simulink model "solverDiscStatesMultirate"  (R2022b)
settings: Solver=VariableStepDiscrete  StartTime=0.0  StopTime=20  RelTol=1e-3
settings Model: Creator=jrivitus  LastModifiedBy=bensweet
settings SolverCC: AlgebraicLoopSolver=TrustRegion
settings DataIOCC: LimitDataPoints=on  SaveFormat=Array  ReturnWorkspaceOutputs=off
settings OptimizationCC: ExpressionDepthLimit=2147483647  InitFltsAndDblsToZero=on  LifeSpan=inf
settings DebuggingCC: UnconnectedInputMsg=warning  UnconnectedOutputMsg=warning  UnconnectedLineMsg=warning  PregeneratedLibrarySubsystemCodeDiagnostic=none  SFMachineParentedDataDiag=warning
settings HardwareCC: ProdBitPerPointer=32  ProdBitPerSizeT=32  ProdBitPerPtrDiffT=32  ProdLargestAtomicFloat=None  ProdIntDivRoundTo=Undefined  ProdEndianess=Unspecified  ProdWordSize=32  ProdHWDeviceType=32-bit Generic
settings ModelReferenceCC: EnableRefExpFcnMdlSchedulingChecks=on  PropagateSignalLabelsOutOfModel=off
settings SFSimCC: SimUseLocalCustomCode=off
settings RTWCC: RTWUseLocalCustomCode=off  DLArmComputeVersion=19.05
settings CodeAppCC: StateflowObjectComments=on
settings GRTTargetCC: TargetLangStandard=C89/C90 (ANSI)  CombineOutputUpdateFcns=off  GRTInterface=on
settings ConfigComp: CovMetricSettings=dw  CovSaveCumulativeToWorkspaceVar=on  CovSaveSingleToWorkspaceVar=on  CovExternalEMLEnable=off  CovSFcnEnable=off

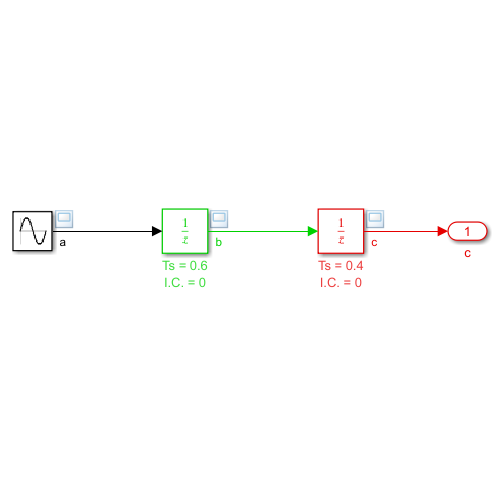
[thumbnail: Simulink's stored preview of the top-level diagram]
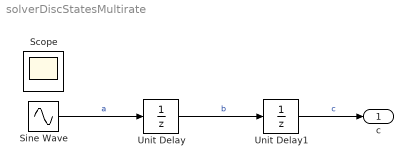
== system solverDiscStatesMultirate ==
  Sine Wave : Sin  SampleTime=0
  Unit Delay : UnitDelay  SampleTime=0.6  HasFrameUpgradeWarning=on
      settings: AttributesFormatString=|
      | Ts = %<SampleTime>
      | I.C. = %<InitialCondition>
  Unit Delay1 : UnitDelay  SampleTime=0.4  HasFrameUpgradeWarning=on
      settings: AttributesFormatString=|
      | Ts = %<SampleTime>
      | I.C. = %<InitialCondition>
  c : Outport  VectorParamsAs1DForOutWhenUnconnected=off
  Scope : Scope
  wires:
  Sine Wave/1 -> Unit Delay/1  "a"
  Unit Delay1/1 -> c/1  "c"
  Unit Delay/1 -> Unit Delay1/1  "b"
